simulink model "G474_SpeedLoop"  (R2024a)
settings: Solver=FixedStepAuto  StartTime=0.0  StopTime=10  FixedStep=0.0001  RelTol=1e-3
values from neighbouring files (symbols this model uses):
  currentKi = 1.5    [ACM4010.sldd]
  currentKp = 3.5    [ACM4010.sldd]
  flux = 0.006    [ACM4010.sldd]
  J = 6.0E-6    [ACM4010.sldd]
  Ki_spd = 0.06    [ACM4010.sldd]
  Kp_spd = 0.025    [ACM4010.sldd]
  Ld = 0.0002    [ACM4010.sldd]
  Lq = 0.0002    [ACM4010.sldd]
  Pn = 5.0    [ACM4010.sldd]
undefined symbols (not defined in the file or in its folder): DiscIntNeverNeededParam, sigbuilder_block
libraries: mcbcontrolslib x6, slpidlib x3, mcbplantlib x1, simulink x1, autolibpmsminterior x1
settings Model: DataDictionary=ACM4010.sldd  Creator=zizhong  LastModifiedBy=zizhong
settings OptimizationCC: DefaultParameterBehavior=Inlined  UseDivisionForNetSlopeComputation=on  GainParamInheritBuiltInType=on  UseFloatMulNetSlope=on  InlineInvariantSignals=on  PassReuseOutputArgsAs=Individual arguments  ZeroExternalMemoryAtStartup=off  ZeroInternalMemoryAtStartup=off  NoFixptDivByZeroProtection=on  EfficientFloat2IntCast=on  LifeSpan=1  MaxStackSize=64  OptimizeBlockOrder=speed  DifferentSizesBufferReuse=on  EfficientTunableParamExpr=on
settings DebuggingCC: ParameterTunabilityLossMsg=error
settings HardwareCC: ProdBitPerPointer=32  ProdBitPerSizeT=32  ProdBitPerPtrDiffT=32  ProdLargestAtomicInteger=Long  ProdLargestAtomicFloat=Double  ProdWordSize=32  ProdLongLongMode=on  ProdHWDeviceType=ARM Compatible->ARM Cortex-M
settings SFSimCC: MATLABDynamicMemAlloc=off  SimTargetLang=C++
settings RTWCC: Description=Embedded Coder  SystemTargetFile=ert.tlc  TemplateMakefile=ert_default_tmf  Toolchain=GNU Tools for ARM Embedded Processors
settings CodeAppCC: ForceParamTrailComments=on  IgnoreCustomStorageClasses=off  OperatorAnnotations=on  SimulinkDataObjDesc=on  SFDataObjDesc=on  CustomSymbolStrGlobalVar=rt$N$M  CustomSymbolStrType=$N$M  CustomSymbolStrFcn=$N$M$F  CustomSymbolStrMacro=$N$M  InsertBlockDesc=on
settings ERTTargetCC: TargetLangStandard=C99 (ISO)  CodeReplacementLibrary=ARM Cortex-M  IncludeMdlTerminateFcn=off  CombineSignalStateStructs=on  SupportComplex=off  SupportNonInlinedSFcns=on  ExtModeTransport=3  ExtModeStaticAlloc=on  ExtModeStaticAllocSize=2048  ExtModeMexFile=ext_xcp  ExtModeIntrfLevel=Level2 - Open  InlinedParameterPlacement=NonHierarchical  ERTCustomFileTemplate=example_file_process.tlc  ERTFilePackagingFormat=CompactWithDataFile

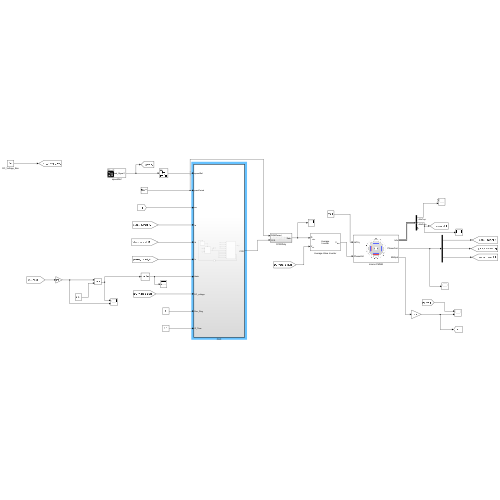
[thumbnail: Simulink's stored preview of the top-level diagram]
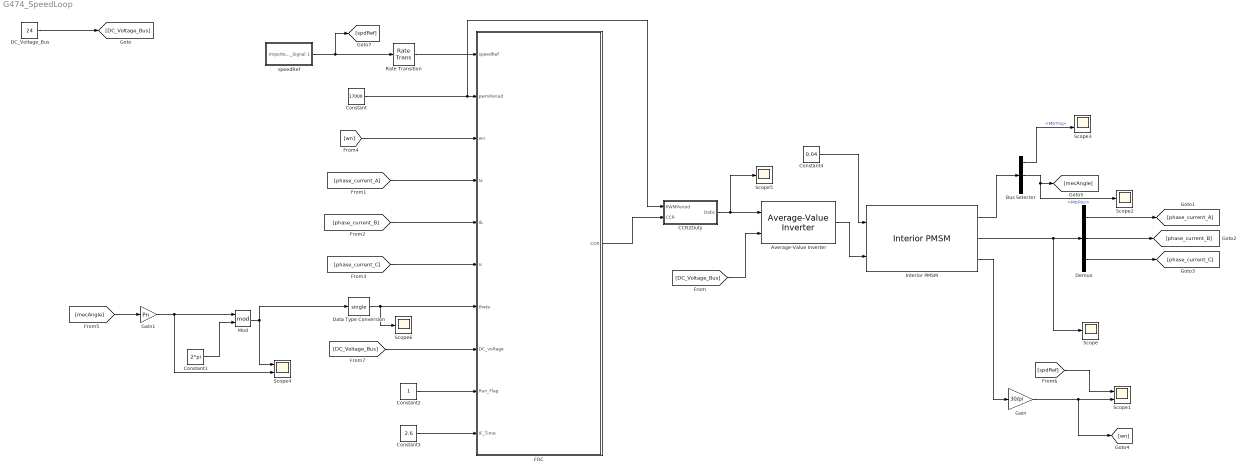
== system G474_SpeedLoop ==
  Average-Value Inverter : mcbplantlib/Average-Value Inverter
      settings: LibrarySourceBlock=mcblib/Electrical Systems/Inverters/Average-Value Inverter
  Bus Selector : BusSelector  OutputSignals=MtrTrq,MtrPos,PwrInfo.PwrTrnsfrd
  CCR2Duty : Subsystem
  Constant : Constant  Value=17000
  Constant1 : Constant  Value=2*pi
  Constant2 : Constant
  Constant3 : Constant  Value=2.6  OutDataTypeStr=single
  Constant4 : Constant  Value=0.04
  DC_Voltage_Bus : Constant  Value=24
  Data Type Conversion : DataTypeConversion  OutDataTypeStr=single  SaturateOnIntegerOverflow=off  RndMeth=Floor
  Demux : Demux  Outputs=3
  FOC : Subsystem  TreatAsAtomicUnit=on
      settings: MinAlgLoopOccurrences=on
  Gain : Gain  Gain=30/pi
  Gain1 : Gain  Gain=Pn
  Interior PMSM : autolibpmsminterior/Interior PMSM  port_config=Torque  sim_type=Discrete  Ts=0.0001  P=Pn  Rs=Rs  Ldq=[Ld Lq]  KConstText=Permanent flux linkage constant (lambda_pm):  lambda_pm=flux  Ke=159.9771  mechanical=[J,0.924e-4,0]  idq0=[0 0]  theta_init=0  omega_init=0  KConst=flux  lambda_pm_calc=flux  Kt=0.07  RefBlkName='autolibpmsminterior/Interior PMSM'  aMode=5
      settings: LibrarySourceBlock=mcblib/Electrical Systems/Motors/Interior PMSM
  Mod : Math  Operator=mod
  Rate Transition : RateTransition
  Scope{,2,5..6} (4 alike) : Scope
  Scope1 : Scope  NumInputPorts=2
  Scope3 : Scope  NumInputPorts=2
  Scope4 : Scope  NumInputPorts=2
  speedRef : Subsystem  Tag=STV Subsys  LoadFcn=sigbuilder_block('load');  StartFcn=sigbuilder_block('start');  StopFcn=sigbuilder_block('stop');  ClipboardFcn=sigbuilder_block('clipboard');  mask(Sigbuilder block){tuvar=[0:10]}
      mask help: Simulink:masks:SigbuilderBlock_MD
      mask init:
      | if ~strcmp(get_param(bdroot(gcbh),'SimulationStatus'),'stopped') tuvar = sigbuilder_block('maskInit'); end
      settings: CopyFcn=sigbuilder_block('copy');  DeleteFcn=sigbuilder_block('delete');  ModelCloseFcn=sigbuilder_block('modelClose');  PreSaveFcn=sigbuilder_block('preSave');  PauseFcn=sigbuilder_block('pause');  ContinueFcn=sigbuilder_block('continue');  NameChangeFcn=sigbuilder_block('namechange');  OpenFcn=sigbuilder_block('open',[5.5 36 1269 593 ]);  CloseFcn=sigbuilder_block('close');
      mask Display: plot(0, 0, 100, 100,[2, 2, 32, 32, 2], [68, 8, 8, 68, 68],[32, 2], [38, 38], [32, 19, 2],[53, 60, 44], [32, 17, 17, 2],[16, 16, 31, 31]);txt = getActiveGroup(gcbh);text(2, 100, txt,'verticalAlignment', 'top');
  wires:
  Demux/3 -> [phase_current_C]
  Rate Transition/1 -> FOC/1(speedRef)
  Interior PMSM/2 -> Scope/1, Demux/1
  Average-Value Inverter/1 -> Interior PMSM/2
  CCR2Duty/1(Dabc) -> Scope5/1, Average-Value Inverter/1
  [DC_Voltage_Bus] -> Average-Value Inverter/2
  Bus Selector/1 -> Scope3/2  "<MtrTrq>"
  Gain1/1 -> Scope4/2, Mod/1
  Interior PMSM/3 -> Gain/1
  Interior PMSM/1 -> Bus Selector/1
  Constant1/1 -> Mod/2
  [wn] -> FOC/3(wn)
  Demux/1 -> [phase_current_A]
  speedRef/1(Imported_Signal 1) -> Rate Transition/1, [spdRef]
  [mecAngle] -> Gain1/1
  [phase_current_C] -> FOC/6(Ic)
  Constant/1 -> CCR2Duty/1(PWMPeriod), FOC/2(pwmPeriod)
  [phase_current_A] -> FOC/4(Ia)
  Gain/1 -> [wn], Scope1/2
  Mod/1 -> Scope4/1, Data Type Conversion/1
  [phase_current_B] -> FOC/5(Ib)
  Bus Selector/2 -> Scope2/1, [mecAngle]  "<MtrPos>"
  Demux/2 -> [phase_current_B]
  DC_Voltage_Bus/1 -> [DC_Voltage_Bus]
  [DC_Voltage_Bus] -> FOC/8(DC_voltage)
  Constant2/1 -> FOC/9(Run_Flag)
  FOC/1(CCR) -> CCR2Duty/2(CCR)
  Constant3/1 -> FOC/10(IF_Time)
  Data Type Conversion/1 -> Scope6/1, FOC/7(theta)
  [spdRef] -> Scope1/1
  Constant4/1 -> Interior PMSM/1

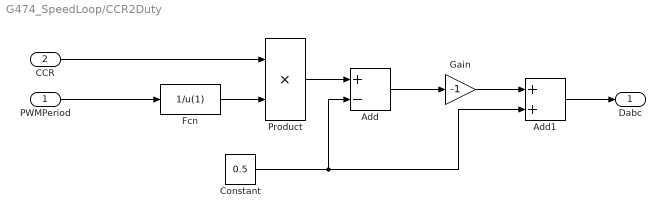
== system G474_SpeedLoop/CCR2Duty ==
  PWMPeriod : Inport
  CCR : Inport  Port=2
  Add : Sum  Inputs=+-
  Add1 : Sum
  Constant : Constant  Value=0.5
  Fcn : Fcn  Expr=1/u(1)
  Gain : Gain  Gain=-1
  Product : Product
  Dabc : Outport
  wires:
  PWMPeriod/1 -> Fcn/1
  Fcn/1 -> Product/2
  CCR/1 -> Product/1
  Product/1 -> Add/1
  Constant/1 -> Add1/2, Add/2
  Add/1 -> Gain/1
  Gain/1 -> Add1/1
  Add1/1 -> Dabc/1

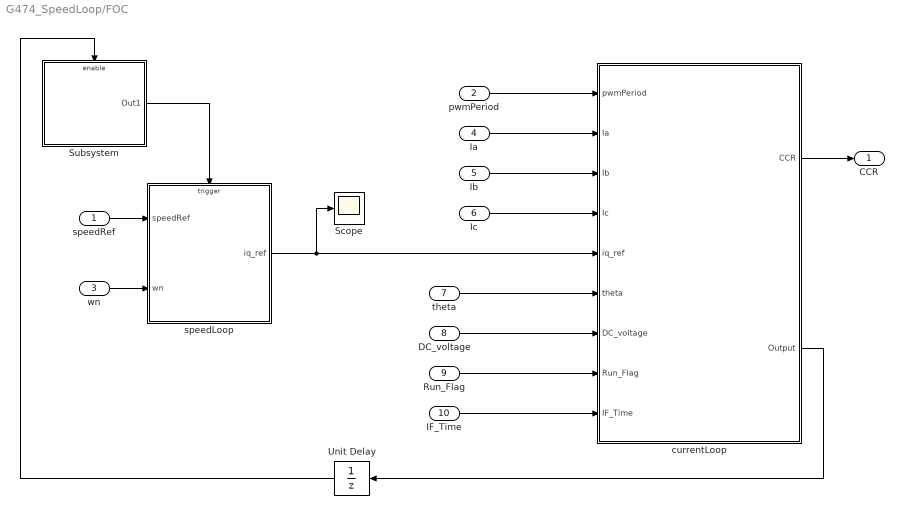
== system G474_SpeedLoop/FOC ==
  speedRef : Inport
  pwmPeriod : Inport  Port=2
  wn : Inport  Port=3
  Ia : Inport  Port=4
  Ib : Inport  Port=5
  Ic : Inport  Port=6
  theta : Inport  Port=7
  DC_voltage : Inport  Port=8
  Run_Flag : Inport  Port=9
  IF_Time : Inport  Port=10
  Scope : Scope
  Subsystem : Subsystem
  Unit Delay : UnitDelay  SampleTime=-1  HasFrameUpgradeWarning=on
  currentLoop : Subsystem  TreatAsAtomicUnit=on
      settings: MinAlgLoopOccurrences=on
  speedLoop : Subsystem  TreatAsAtomicUnit=on
      settings: MinAlgLoopOccurrences=on
  CCR : Outport
  wires:
  pwmPeriod/1 -> currentLoop/1(pwmPeriod)
  Ia/1 -> currentLoop/2(Ia)
  Ib/1 -> currentLoop/3(Ib)
  Ic/1 -> currentLoop/4(Ic)
  theta/1 -> currentLoop/6(theta)
  DC_voltage/1 -> currentLoop/7(DC_voltage)
  Run_Flag/1 -> currentLoop/8(Run_Flag)
  IF_Time/1 -> currentLoop/9(IF_Time)
  currentLoop/1(CCR) -> CCR/1
  speedRef/1 -> speedLoop/1(speedRef)
  wn/1 -> speedLoop/2(wn)
  speedLoop/1(iq_ref) -> currentLoop/5(iq_ref), Scope/1
  currentLoop/2(Output) -> Unit Delay/1
  Unit Delay/1 -> Subsystem/Enable
  Subsystem/1(Out1) -> speedLoop/Trigger

== system G474_SpeedLoop/speedRef ==
  Demux : Demux  Tag=STV Demux  Outputs=1
      settings: DisplayOption=none
  FromWs : FromWorkspace  Tag=STV FromWs  VariableName=tuvar
      SigBuilderData=|
      | common.afterFinalStr = 'Extrapolate'
      | common.sampleTime = 0
      | dataSet.timeRange = [0 10]
      | dataSet.name = 'Sheet1'
      | sbobj.Groups.Name = 'Sheet1'
      | sbobj.Groups.Signals.Name = 'Imported_Signal 1'
      | sbobj.Groups.Signals.XData = [0 1 2 3 4 5 5.96 7 8 9 10]
      | sbobj.Groups.Signals.YData = [500 500 500 500 934 5000 5170 5210 5200 5220 5210]
  Imported_Signal 1 : Outport  Tag=STV Outport
  wires:
  Demux/1 -> Imported_Signal 1/1
  FromWs/1 -> Demux/1

== system G474_SpeedLoop/FOC/Subsystem ==
  Enable : EnablePort
  Function-Call Generator : simulink/Ports & Subsystems/Function-Call Generator  sample_time=1e-3  numberOfIterations=1  DisallowWideOutput=off
  Out1 : Outport
  wires:
  Function-Call Generator/1 -> Out1/1

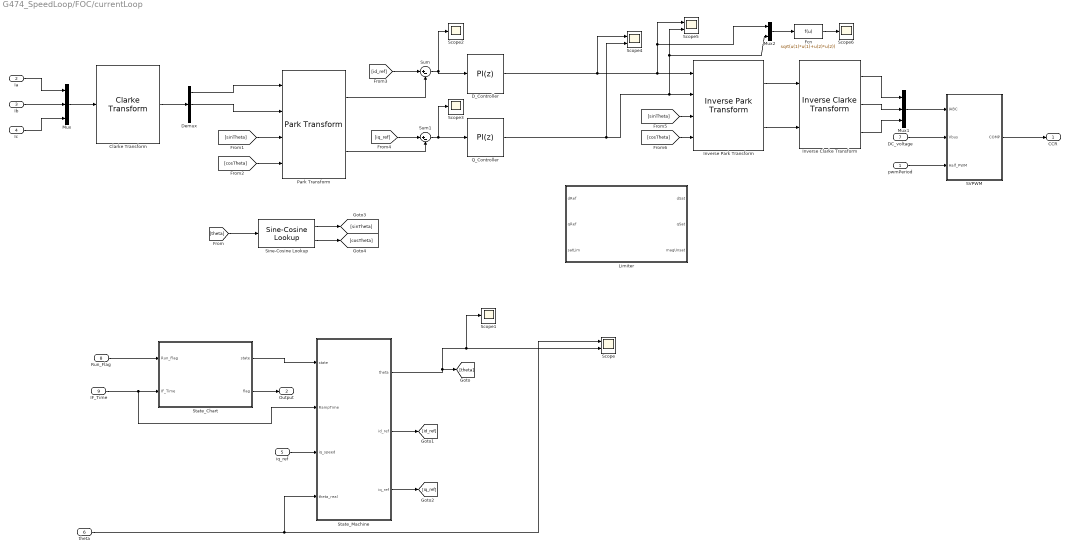
== system G474_SpeedLoop/FOC/currentLoop ==
  pwmPeriod : Inport
  Ia : Inport  Port=2
  Ib : Inport  Port=3
  Ic : Inport  Port=4
  iq_ref : Inport  Port=5
  theta : Inport  Port=6
  DC_voltage : Inport  Port=7
  Run_Flag : Inport  Port=8
  IF_Time : Inport  Port=9
  Clarke Transform : mcbcontrolslib/Clarke Transform  VariantControl=Variant2  PhaseInput=Three inputs  EnPowerInv=off
      settings: LibrarySourceBlock=mcbhdllib/Controls/Math Transforms/Clarke Transform
  D_Controller : slpidlib/PID Controller  Controller=PI  Form=Parallel  TimeDomain=Discrete-time  UseExternalTs=off  SampleTime=-1  IntegratorMethod=Forward Euler  FilterMethod=Forward Euler  ControllerParametersSource=internal  P=currentKp  I=currentKi  UseKiTs=off  D=0  UseExternalDerivativeSource=off  N=100  UseFilter=on  TunerSelectOption=Transfer Function Based (PID Tuner App)  InitialConditionSource=internal  InitialConditionForIntegrator=0  InitialConditionForFilter=0  DifferentiatorICPrevScaledInput=0  ExternalReset=none  TrackingMode=off  Kt=1  LimitOutput=on  SatLimitsSource=internal  UpperSaturationLimit=12  LowerSaturationLimit=-12  LinearizeAsGain=on  AntiWindupMode=clamping  Kb=1  LimitIntegrator=off  UpperIntegratorSaturationLimit=inf  LowerIntegratorSaturationLimit=-inf  PGainOutDataTypeStr=single  PProdOutDataTypeStr=single  POutMin=[]  POutMax=[]  IGainOutDataTypeStr=int16  IProdOutDataTypeStr=int16  IOutMin=[]  IOutMax=[]  DOutMin=[]  DOutMax=[]  NOutMin=[]  NOutMax=[]  SumOutDataTypeStr=single  SumOutMin=[]  SumOutMax=[]  SaturationOutDataTypeStr=single  SaturationOutMin=[]  SaturationOutMax=[]  PParamMin=[]  PParamMax=[]  IParamMin=[]  IParamMax=[]  DParamMin=[]  DParamMax=[]  NParamMin=[]  NParamMax=[]  KbParamMin=[]  KbParamMax=[]  KtParamMin=[]  KtParamMax=[]  KbOutMin=[]  KbOutMax=[]  KtOutMin=[]  KtOutMax=[]  IntegratorOutMin=[]  IntegratorOutMax=[]  FilterOutMin=[]  FilterOutMax=[]  SumI1OutMin=[]  SumI1OutMax=[]  SumI2OutMin=[]  SumI2OutMax=[]  SumI3OutMin=[]  SumI3OutMax=[]  SumI4OutMin=[]  SumI4OutMax=[]  SumDOutMin=[]  SumDOutMax=[]  DifferentiatorOutMin=[]  DifferentiatorOutMax=[]  FilterDiffOutCoefMin=[]  FilterDiffOutCoefMax=[]  ReciprocalOutMin=[]  ReciprocalOutMax=[]  SumDenOutMin=[]  SumDenOutMax=[]  SumNumOutMin=[]  SumNumOutMax=[]  DivideOutMin=[]  DivideOutMax=[]  UdiffTsProdOutMin=[]  UdiffTsProdOutMax=[]  NTsProdOutMin=[]  NTsProdOutMax=[]  UintegralTsProdOutMin=[]  UintegralTsProdOutMax=[]  UngainTsProdOutMin=[]  UngainTsProdOutMax=[]  ClampingZeroOutDataTypeStr=Inherit: Inherit via back propagation  ClampingZeroOutMin=[]  ClampingZeroOutMax=[]  FilterDenConstantOutDataTypeStr=Inherit: Inherit via back propagation  FilterDenConstantOutMin=[]  FilterDenConstantOutMax=[]  PCopyOutDataTypeStr=Inherit: Inherit via back propagation  PCopyOutMin=[]  PCopyOutMax=[]  NCopyOutDataTypeStr=Inherit: Inherit via back propagation  NCopyOutMin=[]  NCopyOutMax=[]  IntegratorContinuousStateAttributes=''  IntegratorStateMustResolveToSignalObject=off  IntegratorRTWStateStorageClass=Auto  FilterContinuousStateAttributes=''  FilterStateMustResolveToSignalObject=off  FilterRTWStateStorageClass=Auto  ParallelPVariant=InternalParameters  IdealPVariant=Disabled  IVariant=InternalParameters  DVariant=Disabled  IntegratorVariant=Discrete  SatVariant=Enabled  AWVariant=DiscClampingParallel  PCopyVariant=Disabled  TRVariant=Disabled  FdbkBlocksVariant=Forward  IdealPFdbkVariant=Disabled  SatFdbkVariant=Disabled  DerivativeFilterVariant=Disabled  NVariant=Disabled  NCopyVariant=Disabled_SignalSpec  FilterICVariant=Disabled  IntegratorICVariant=InternalICs  ExternalResetVariant=Disabled  TRSumVariant=Passthrough  SumFdbkVariant=Disabled  SumVariant=Sum_PI  TsampFilterVariant=InternalTs  TsampNgainVariant=Passthrough  TsampIntegralVariant=Disabled_SignalSpec  ExternalSaturationOutDataTypeStr=Inherit: Same as second input  DerivativeSourceVariant=Disabled
  Demux : Demux  Outputs=3
  Fcn : Fcn  Expr=sqrt(u(1)*u(1)+u(2)*u(2))
  Inverse Clarke Transform : mcbcontrolslib/Inverse Clarke Transform  PhaseInput=Two inputs  EnPowerInv=off
      settings: LibrarySourceBlock=mcbhdllib/Controls/Math Transforms/Inverse Clarke Transform
  Inverse Park Transform : mcbcontrolslib/Inverse Park Transform  PhaseInput=Two inputs  AxisAlignment=D-axis  ThetaInput=Sine and Cosine electrical position  AngleInput=Per-unit  N_points=1024
      settings: LibrarySourceBlock=mcbhdllib/Controls/Math Transforms/Inverse Park Transform
  Limiter : Subsystem
  Mux : Mux  Inputs=3
  Mux1 : Mux  Inputs=3
  Mux2 : Mux  Inputs=2
  Park Transform : mcbcontrolslib/Park Transform  PhaseInput=Two inputs  AxisAlignment=D-axis  ThetaInput=Sine and Cosine electrical position  AngleInput=Per-unit  N_points=1024
      settings: LibrarySourceBlock=mcbhdllib/Controls/Math Transforms/Park Transform
  Q_Controller : slpidlib/PID Controller  Controller=PI  Form=Parallel  TimeDomain=Discrete-time  UseExternalTs=off  SampleTime=-1  IntegratorMethod=Forward Euler  FilterMethod=Forward Euler  ControllerParametersSource=internal  P=currentKp  I=currentKi  UseKiTs=off  D=0  UseExternalDerivativeSource=off  N=100  UseFilter=on  TunerSelectOption=Transfer Function Based (PID Tuner App)  InitialConditionSource=internal  InitialConditionForIntegrator=0  InitialConditionForFilter=0  DifferentiatorICPrevScaledInput=0  ExternalReset=none  TrackingMode=off  Kt=1  LimitOutput=on  SatLimitsSource=internal  UpperSaturationLimit=12  LowerSaturationLimit=-12  LinearizeAsGain=on  AntiWindupMode=clamping  Kb=1  LimitIntegrator=off  UpperIntegratorSaturationLimit=inf  LowerIntegratorSaturationLimit=-inf  PGainOutDataTypeStr=single  PProdOutDataTypeStr=single  POutMin=[]  POutMax=[]  IGainOutDataTypeStr=int16  IProdOutDataTypeStr=int16  IOutMin=[]  IOutMax=[]  DOutMin=[]  DOutMax=[]  NOutMin=[]  NOutMax=[]  SumOutDataTypeStr=single  SumOutMin=[]  SumOutMax=[]  SaturationOutDataTypeStr=single  SaturationOutMin=[]  SaturationOutMax=[]  PParamMin=[]  PParamMax=[]  IParamMin=[]  IParamMax=[]  DParamMin=[]  DParamMax=[]  NParamMin=[]  NParamMax=[]  KbParamMin=[]  KbParamMax=[]  KtParamMin=[]  KtParamMax=[]  KbOutMin=[]  KbOutMax=[]  KtOutMin=[]  KtOutMax=[]  IntegratorOutMin=[]  IntegratorOutMax=[]  FilterOutMin=[]  FilterOutMax=[]  SumI1OutMin=[]  SumI1OutMax=[]  SumI2OutMin=[]  SumI2OutMax=[]  SumI3OutMin=[]  SumI3OutMax=[]  SumI4OutMin=[]  SumI4OutMax=[]  SumDOutMin=[]  SumDOutMax=[]  DifferentiatorOutMin=[]  DifferentiatorOutMax=[]  FilterDiffOutCoefMin=[]  FilterDiffOutCoefMax=[]  ReciprocalOutMin=[]  ReciprocalOutMax=[]  SumDenOutMin=[]  SumDenOutMax=[]  SumNumOutMin=[]  SumNumOutMax=[]  DivideOutMin=[]  DivideOutMax=[]  UdiffTsProdOutMin=[]  UdiffTsProdOutMax=[]  NTsProdOutMin=[]  NTsProdOutMax=[]  UintegralTsProdOutMin=[]  UintegralTsProdOutMax=[]  UngainTsProdOutMin=[]  UngainTsProdOutMax=[]  ClampingZeroOutDataTypeStr=Inherit: Inherit via back propagation  ClampingZeroOutMin=[]  ClampingZeroOutMax=[]  FilterDenConstantOutDataTypeStr=Inherit: Inherit via back propagation  FilterDenConstantOutMin=[]  FilterDenConstantOutMax=[]  PCopyOutDataTypeStr=Inherit: Inherit via back propagation  PCopyOutMin=[]  PCopyOutMax=[]  NCopyOutDataTypeStr=Inherit: Inherit via back propagation  NCopyOutMin=[]  NCopyOutMax=[]  IntegratorContinuousStateAttributes=''  IntegratorStateMustResolveToSignalObject=off  IntegratorRTWStateStorageClass=Auto  FilterContinuousStateAttributes=''  FilterStateMustResolveToSignalObject=off  FilterRTWStateStorageClass=Auto  ParallelPVariant=InternalParameters  IdealPVariant=Disabled  IVariant=InternalParameters  DVariant=Disabled  IntegratorVariant=Discrete  SatVariant=Enabled  AWVariant=DiscClampingParallel  PCopyVariant=Disabled  TRVariant=Disabled  FdbkBlocksVariant=Forward  IdealPFdbkVariant=Disabled  SatFdbkVariant=Disabled  DerivativeFilterVariant=Disabled  NVariant=Disabled  NCopyVariant=Disabled_SignalSpec  FilterICVariant=Disabled  IntegratorICVariant=InternalICs  ExternalResetVariant=Disabled  TRSumVariant=Passthrough  SumFdbkVariant=Disabled  SumVariant=Sum_PI  TsampFilterVariant=InternalTs  TsampNgainVariant=Passthrough  TsampIntegralVariant=Disabled_SignalSpec  ExternalSaturationOutDataTypeStr=Inherit: Same as second input  DerivativeSourceVariant=Disabled
  SVPWM : Subsystem  TreatAsAtomicUnit=on
      settings: MinAlgLoopOccurrences=on
  Scope : Scope  NumInputPorts=2
  Scope{1..3,6} (4 alike) : Scope
  Scope4 : Scope  NumInputPorts=2
  Scope5 : Scope  NumInputPorts=2
  Sine-Cosine Lookup : mcbcontrolslib/Sine-Cosine Lookup  AngleInput=Radians  N_points=1024  DatatypeInput=Inherit from input  Datatype=single
      settings: LibrarySourceBlock=mcblib/Controls/Math Transforms/Sine-Cosine Lookup
  State_Chart : Stateflow chart  TreatAsAtomicUnit=on
  State_Machine : Subsystem  TreatAsAtomicUnit=on
      settings: MinAlgLoopOccurrences=on
  Sum : Sum  Inputs=|+-
  Sum1 : Sum  Inputs=|+-
  CCR : Outport
  Output : Outport  Port=2
  wires:
  State_Chart/2(flag) -> Output/1
  Run_Flag/1 -> State_Chart/1(Run_Flag)
  IF_Time/1 -> State_Machine/2(RampTime), State_Chart/2(IF_Time)
  State_Machine/1(theta) -> Scope1/1, Scope/2, [theta]
  Ib/1 -> Mux/2
  [theta] -> Sine-Cosine Lookup/1
  DC_voltage/1 -> SVPWM/2(Vbus)
  Sine-Cosine Lookup/1 -> [sinTheta]
  Clarke Transform/1 -> Demux/1
  State_Chart/1(state) -> State_Machine/1(state)
  Ia/1 -> Mux/1
  Demux/1 -> Park Transform/1
  Inverse Clarke Transform/2 -> Mux1/2
  State_Machine/3(iq_ref) -> [iq_ref]
  Park Transform/2 -> Sum1/2
  Inverse Clarke Transform/3 -> Mux1/3
  [id_ref] -> Sum/1
  Sum/1 -> D_Controller/1, Scope2/1
  SVPWM/1(COMP) -> CCR/1
  Sum1/1 -> Scope3/1, Q_Controller/1
  theta/1 -> State_Machine/4(theta_real), Scope/1
  [sinTheta] -> Inverse Park Transform/3
  [sinTheta] -> Park Transform/3
  Inverse Park Transform/1 -> Inverse Clarke Transform/1
  Mux1/1 -> SVPWM/1(IABC)
  Mux/1 -> Clarke Transform/1
  [cosTheta] -> Park Transform/4
  State_Machine/2(id_ref) -> [id_ref]
  D_Controller/1 -> Scope4/1, Scope5/1, Mux2/1, Inverse Park Transform/1
  Q_Controller/1 -> Scope4/2, Scope5/2, Mux2/2, Inverse Park Transform/2
  Demux/2 -> Park Transform/2
  Sine-Cosine Lookup/2 -> [cosTheta]
  Inverse Park Transform/2 -> Inverse Clarke Transform/2
  [cosTheta] -> Inverse Park Transform/4
  Ic/1 -> Mux/3
  Inverse Clarke Transform/1 -> Mux1/1
  [iq_ref] -> Sum1/1
  pwmPeriod/1 -> SVPWM/3(Half_PWM)
  Park Transform/1 -> Sum/2
  iq_ref/1 -> State_Machine/3(iq_speed)
  Mux2/1 -> Fcn/1
  Fcn/1 -> Scope6/1

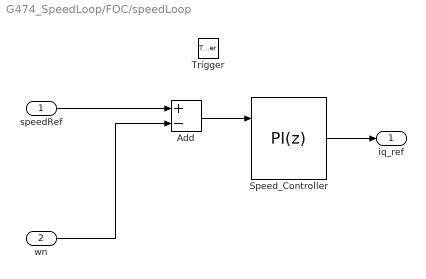
== system G474_SpeedLoop/FOC/speedLoop ==
  speedRef : Inport
  wn : Inport  Port=2
  Trigger : TriggerPort  TriggerType=function-call  VariantControl=(inherit)  PortDimensions=1
  Add : Sum  Inputs=+-
  Speed_Controller : slpidlib/PID Controller  Controller=PI  Form=Parallel  TimeDomain=Discrete-time  UseExternalTs=off  SampleTime=-1  IntegratorMethod=Forward Euler  FilterMethod=Forward Euler  ControllerParametersSource=internal  P=Kp_spd  I=Ki_spd  UseKiTs=off  D=0  UseExternalDerivativeSource=off  N=100  UseFilter=on  TunerSelectOption=Transfer Function Based (PID Tuner App)  InitialConditionSource=internal  InitialConditionForIntegrator=0  InitialConditionForFilter=0  DifferentiatorICPrevScaledInput=0  ExternalReset=rising  TrackingMode=off  Kt=1  LimitOutput=on  SatLimitsSource=internal  UpperSaturationLimit=10  LowerSaturationLimit=-10  LinearizeAsGain=on  AntiWindupMode=clamping  Kb=1  LimitIntegrator=off  UpperIntegratorSaturationLimit=100  LowerIntegratorSaturationLimit=-100  PGainOutDataTypeStr=single  PProdOutDataTypeStr=single  POutMin=[]  POutMax=[]  IGainOutDataTypeStr=int16  IProdOutDataTypeStr=int16  IOutMin=[]  IOutMax=[]  DOutMin=[]  DOutMax=[]  NOutMin=[]  NOutMax=[]  SumOutDataTypeStr=single  SumOutMin=[]  SumOutMax=[]  SaturationOutDataTypeStr=single  SaturationOutMin=[]  SaturationOutMax=[]  PParamMin=[]  PParamMax=[]  IParamMin=[]  IParamMax=[]  DParamMin=[]  DParamMax=[]  NParamMin=[]  NParamMax=[]  KbParamMin=[]  KbParamMax=[]  KtParamMin=[]  KtParamMax=[]  KbOutMin=[]  KbOutMax=[]  KtOutMin=[]  KtOutMax=[]  IntegratorOutMin=[]  IntegratorOutMax=[]  FilterOutMin=[]  FilterOutMax=[]  SumI1OutMin=[]  SumI1OutMax=[]  SumI2OutMin=[]  SumI2OutMax=[]  SumI3OutMin=[]  SumI3OutMax=[]  SumI4OutMin=[]  SumI4OutMax=[]  SumDOutMin=[]  SumDOutMax=[]  DifferentiatorOutMin=[]  DifferentiatorOutMax=[]  FilterDiffOutCoefMin=[]  FilterDiffOutCoefMax=[]  ReciprocalOutMin=[]  ReciprocalOutMax=[]  SumDenOutMin=[]  SumDenOutMax=[]  SumNumOutMin=[]  SumNumOutMax=[]  DivideOutMin=[]  DivideOutMax=[]  UdiffTsProdOutMin=[]  UdiffTsProdOutMax=[]  NTsProdOutMin=[]  NTsProdOutMax=[]  UintegralTsProdOutMin=[]  UintegralTsProdOutMax=[]  UngainTsProdOutMin=[]  UngainTsProdOutMax=[]  ClampingZeroOutDataTypeStr=Inherit: Inherit via back propagation  ClampingZeroOutMin=[]  ClampingZeroOutMax=[]  FilterDenConstantOutDataTypeStr=Inherit: Inherit via back propagation  FilterDenConstantOutMin=[]  FilterDenConstantOutMax=[]  PCopyOutDataTypeStr=Inherit: Inherit via back propagation  PCopyOutMin=[]  PCopyOutMax=[]  NCopyOutDataTypeStr=Inherit: Inherit via back propagation  NCopyOutMin=[]  NCopyOutMax=[]  IntegratorContinuousStateAttributes=''  IntegratorStateMustResolveToSignalObject=off  IntegratorRTWStateStorageClass=Auto  FilterContinuousStateAttributes=''  FilterStateMustResolveToSignalObject=off  FilterRTWStateStorageClass=Auto  ParallelPVariant=InternalParameters  IdealPVariant=Disabled  IVariant=InternalParameters  DVariant=Disabled  IntegratorVariant=Discrete  SatVariant=Enabled  AWVariant=DiscClampingParallel  PCopyVariant=Disabled  TRVariant=Disabled  FdbkBlocksVariant=Forward  IdealPFdbkVariant=Disabled  SatFdbkVariant=Disabled  DerivativeFilterVariant=Disabled  NVariant=Disabled  NCopyVariant=Disabled_SignalSpec  FilterICVariant=Disabled  IntegratorICVariant=InternalICs  ExternalResetVariant=ExternalReset  TRSumVariant=Passthrough  SumFdbkVariant=Disabled  SumVariant=Sum_PI  TsampFilterVariant=InternalTs  TsampNgainVariant=Passthrough  TsampIntegralVariant=Disabled_SignalSpec  ExternalSaturationOutDataTypeStr=Inherit: Same as second input  DerivativeSourceVariant=Disabled
  iq_ref : Outport
  wires:
  Speed_Controller/1 -> iq_ref/1
  speedRef/1 -> Add/1
  wn/1 -> Add/2
  Add/1 -> Speed_Controller/1

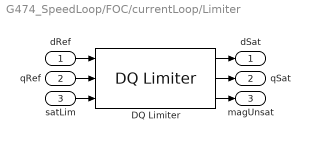
== system G474_SpeedLoop/FOC/currentLoop/Limiter ==
  dRef : Inport
  qRef : Inport  Port=2
  satLim : Inport  Port=3
  DQ Limiter : mcbcontrolslib/DQ Limiter  satMethodInputType=Specify via dialog  satMethodSelected=D-Q equivalence  satLimitInputType=Input port  Vmax=1
      settings: LibrarySourceBlock=mcbhdllib/Controls/Control Reference/DQ Limiter
  dSat : Outport
  qSat : Outport  Port=2
  magUnsat : Outport  Port=3
  wires:
  dRef/1 -> DQ Limiter/1
  DQ Limiter/2 -> qSat/1
  qRef/1 -> DQ Limiter/2
  satLim/1 -> DQ Limiter/3
  DQ Limiter/1 -> dSat/1
  DQ Limiter/3 -> magUnsat/1

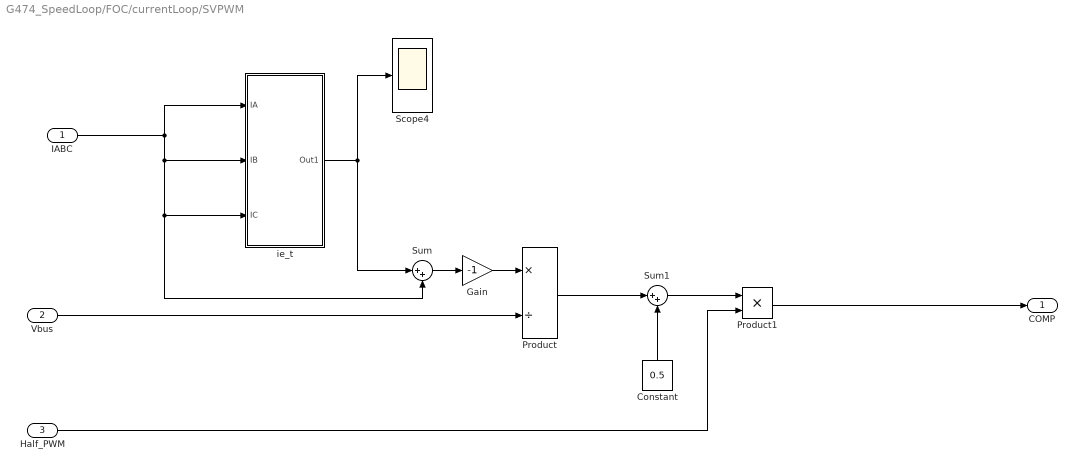
== system G474_SpeedLoop/FOC/currentLoop/SVPWM ==
  IABC : Inport
  Vbus : Inport  Port=2
  Half_PWM : Inport  Port=3
  Constant : Constant  Value=0.5
  Gain : Gain  Gain=-1
  Product : Product  Inputs=*/
  Product1 : Product
  Scope4 : Scope
  Sum : Sum  Inputs=|++
  Sum1 : Sum  Inputs=|++
  ie_t : Subsystem
  COMP : Outport
  wires:
  IABC/1 -> ie_t/3(IC), Sum/2, ie_t/2(IB), ie_t/1(IA)
  Half_PWM/1 -> Product1/2
  Gain/1 -> Product/1
  ie_t/1(Out1) -> Sum/1, Scope4/1
  Sum/1 -> Gain/1
  Sum1/1 -> Product1/1
  Constant/1 -> Sum1/2
  Product/1 -> Sum1/1
  Vbus/1 -> Product/2
  Product1/1 -> COMP/1

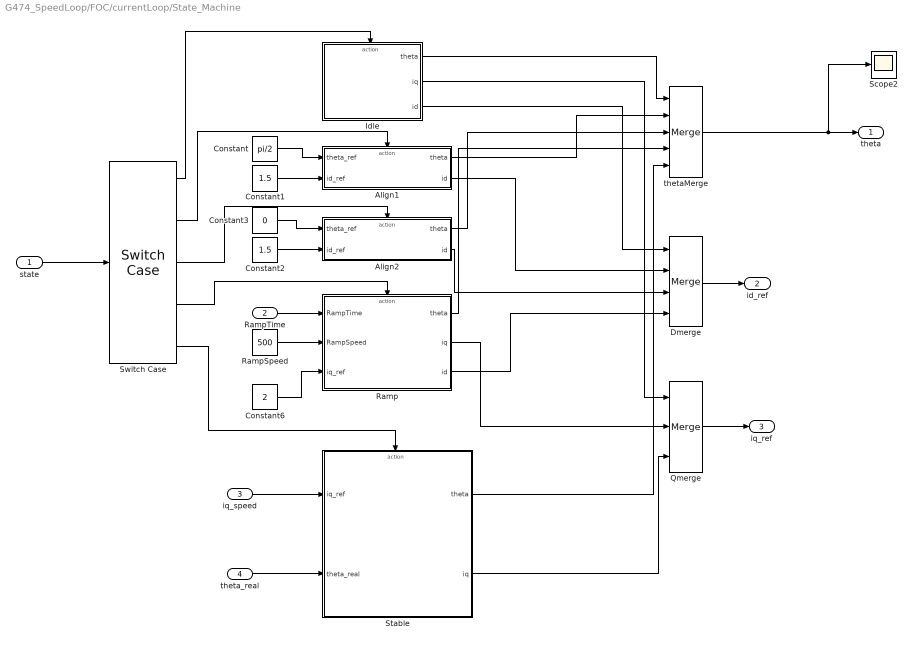
== system G474_SpeedLoop/FOC/currentLoop/State_Machine ==
  state : Inport
  RampTime : Inport  Port=2
  iq_speed : Inport  Port=3
  theta_real : Inport  Port=4
  Align1 : Subsystem  TreatAsAtomicUnit=on
  Align2 : Subsystem  TreatAsAtomicUnit=on
  Constant : Constant  Value=pi/2  OutDataTypeStr=single
  Constant1 : Constant  Value=1.5  OutDataTypeStr=single
  Constant2 : Constant  Value=1.5  OutDataTypeStr=single
  Constant3 : Constant  Value=0  OutDataTypeStr=single
  Constant6 : Constant  Value=2  OutDataTypeStr=single
  Dmerge : Merge  Inputs=4
  Idle : Subsystem  TreatAsAtomicUnit=on
  Qmerge : Merge  Inputs=3
  Ramp : Subsystem  TreatAsAtomicUnit=on
  RampSpeed : Constant  Value=500  OutDataTypeStr=single
  Scope2 : Scope
  Stable : Subsystem  TreatAsAtomicUnit=on
  Switch Case : SwitchCase  CaseConditions={0, 1, 2, 3, 4}  ShowDefaultCase=off
  thetaMerge : Merge  Inputs=5
  theta : Outport
  id_ref : Outport  Port=2
  iq_ref : Outport  Port=3
  wires:
  Align1/2(id) -> Dmerge/2
  Constant/1 -> Align1/1(theta_ref)
  Switch Case/5 -> Stable/Action
  Switch Case/1 -> Idle/Action
  Constant2/1 -> Align2/2(id_ref)
  Stable/2(iq) -> Qmerge/3
  Ramp/2(iq) -> Qmerge/2
  Switch Case/2 -> Align1/Action
  RampSpeed/1 -> Ramp/2(RampSpeed)
  Constant3/1 -> Align2/1(theta_ref)
  Constant6/1 -> Ramp/3(iq_ref)
  Ramp/3(id) -> Dmerge/4
  Align1/1(theta) -> thetaMerge/2
  Dmerge/1 -> id_ref/1
  Idle/3(id) -> Dmerge/1
  Ramp/1(theta) -> thetaMerge/4
  Switch Case/3 -> Align2/Action
  Constant1/1 -> Align1/2(id_ref)
  Align2/2(id) -> Dmerge/3
  Idle/2(iq) -> Qmerge/1
  Switch Case/4 -> Ramp/Action
  Align2/1(theta) -> thetaMerge/3
  Idle/1(theta) -> thetaMerge/1
  RampTime/1 -> Ramp/1(RampTime)
  state/1 -> Switch Case/1
  Qmerge/1 -> iq_ref/1
  thetaMerge/1 -> Scope2/1, theta/1
  Stable/1(theta) -> thetaMerge/5
  iq_speed/1 -> Stable/1(iq_ref)
  theta_real/1 -> Stable/2(theta_real)

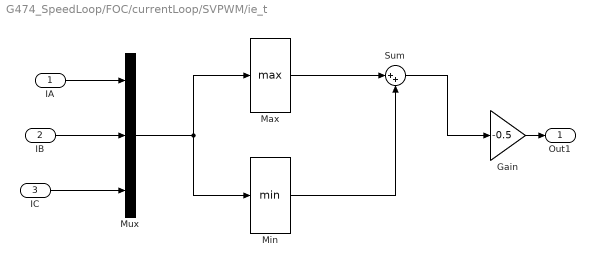
== system G474_SpeedLoop/FOC/currentLoop/SVPWM/ie_t ==
  IA : Inport
  IB : Inport  Port=2
  IC : Inport  Port=3
  Gain : Gain  Gain=-0.5
  Max : MinMax  Function=max
  Min : MinMax
  Mux : Mux  Inputs=3
  Sum : Sum  Inputs=|++
  Out1 : Outport
  wires:
  Max/1 -> Sum/1
  IC/1 -> Mux/3
  Mux/1 -> Min/1, Max/1
  Sum/1 -> Gain/1
  Min/1 -> Sum/2
  IA/1 -> Mux/1
  Gain/1 -> Out1/1
  IB/1 -> Mux/2

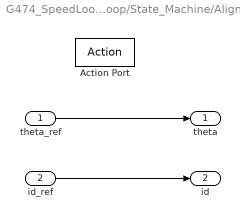
== system G474_SpeedLoop/FOC/currentLoop/State_Machine/Align1 ==
  theta_ref : Inport
  id_ref : Inport  Port=2
  Action Port : ActionPort  ActionPortLabel=case [ 1 ]:
  theta : Outport
  id : Outport  Port=2
  wires:
  theta_ref/1 -> theta/1
  id_ref/1 -> id/1

== system G474_SpeedLoop/FOC/currentLoop/State_Machine/Align2 ==
  theta_ref : Inport
  id_ref : Inport  Port=2
  Action Port : ActionPort  ActionPortLabel=case [ 2 ]:
  theta : Outport
  id : Outport  Port=2
  wires:
  id_ref/1 -> id/1
  theta_ref/1 -> theta/1

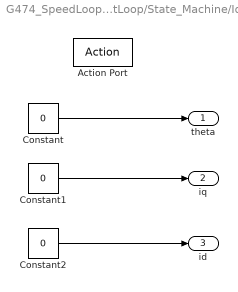
== system G474_SpeedLoop/FOC/currentLoop/State_Machine/Idle ==
  Action Port : ActionPort  ActionPortLabel=case [ 0 ]:
  Constant : Constant  Value=0  OutDataTypeStr=single
  Constant1 : Constant  Value=0  OutDataTypeStr=single
  Constant2 : Constant  Value=0  OutDataTypeStr=single
  theta : Outport
  iq : Outport  Port=2
  id : Outport  Port=3
  wires:
  Constant1/1 -> iq/1
  Constant/1 -> theta/1
  Constant2/1 -> id/1

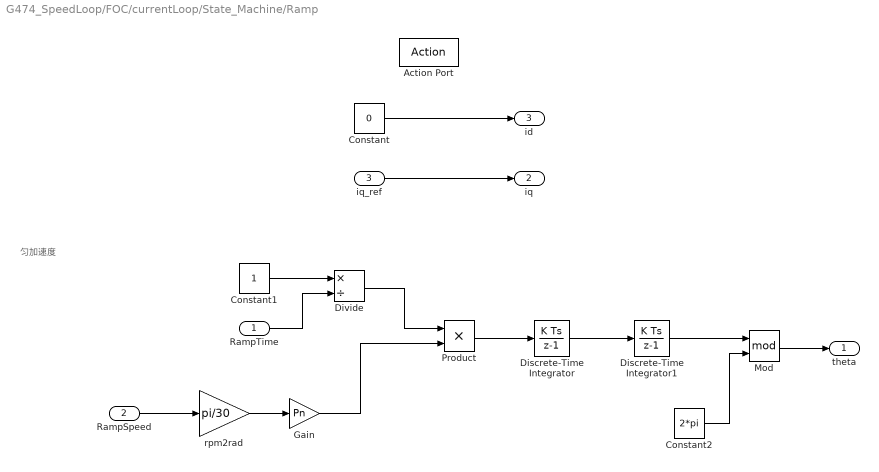
== system G474_SpeedLoop/FOC/currentLoop/State_Machine/Ramp ==
  note: 匀加速度
  RampTime : Inport
  RampSpeed : Inport  Port=2
  iq_ref : Inport  Port=3
  Action Port : ActionPort  ActionPortLabel=case [ 3 ]:
  Constant : Constant  Value=0  OutDataTypeStr=single
  Constant1 : Constant  OutDataTypeStr=single
  Constant2 : Constant  Value=2*pi  OutDataTypeStr=single
  Discrete-Time Integrator : DiscreteIntegrator  SampleTime=-1  ICPrevOutput=DiscIntNeverNeededParam  ICPrevScaledInput=DiscIntNeverNeededParam
  Discrete-Time Integrator1 : DiscreteIntegrator  SampleTime=-1  ICPrevOutput=DiscIntNeverNeededParam  ICPrevScaledInput=DiscIntNeverNeededParam
  Divide : Product  Inputs=*/
  Gain : Gain  Gain=Pn
  Mod : Math  Operator=mod
  Product : Product
  rpm2rad : Gain  Gain=pi/30
  theta : Outport
  iq : Outport  Port=2
  id : Outport  Port=3
  wires:
  Constant/1 -> id/1
  iq_ref/1 -> iq/1
  RampSpeed/1 -> rpm2rad/1
  Constant1/1 -> Divide/1
  RampTime/1 -> Divide/2
  Divide/1 -> Product/1
  rpm2rad/1 -> Gain/1
  Product/1 -> Discrete-Time Integrator/1
  Discrete-Time Integrator/1 -> Discrete-Time Integrator1/1
  Mod/1 -> theta/1
  Constant2/1 -> Mod/2
  Gain/1 -> Product/2
  Discrete-Time Integrator1/1 -> Mod/1

== system G474_SpeedLoop/FOC/currentLoop/State_Machine/Stable ==
  iq_ref : Inport
  theta_real : Inport  Port=2
  Action Port : ActionPort  ActionPortLabel=case [ 4 ]:
  theta : Outport
  iq : Outport  Port=2
  wires:
  iq_ref/1 -> iq/1
  theta_real/1 -> theta/1

== stateflow chart G474_SpeedLoop/FOC/currentLoop/State_Chart ==
  state Ramp
    en:
    state = 3;
  state Idle
    en:
    state = 0;
  state First_Align
    en:
    state = 1;
  state Last_Align
    en:
    state = 2;
  state Stablize
    en:
    state = 4;
  Ramp -> (junction 87) [order 3] : [after(IF_Time * 9999,tick)]{flag = 1}
  (default) -> Idle
  Idle -> First_Align : [Run_Flag == 1]
  First_Align -> Last_Align [order 1] : [after(1000,tick)]
  Last_Align -> Ramp [order 1] : [after(1000,tick)]
  Ramp -> Stablize [order 1] : [after(IF_Time * 10000,tick)]
  First_Align -> Idle [order 2] : [Run_Flag == 0]
  Last_Align -> Idle [order 2] : [Run_Flag == 0]
  Ramp -> Idle [order 2] : [Run_Flag == 0]
  Stablize -> Idle : [Run_Flag == 0]
  data: Run_Flag input; state output; IF_Time input; flag output
